simulink model "payment_donation_hcs_2020"  (R2020a)
settings: Solver=VariableStepAuto  StartTime=0.0  StopTime=10.0  RelTol=1e-3
(part 1 of 2)
settings Model: Creator=ayj  LastModifiedBy=ayj
settings DebuggingCC: UnconnectedInputMsg=none  UnconnectedOutputMsg=none  UnconnectedLineMsg=none  SFMachineParentedDataDiag=error

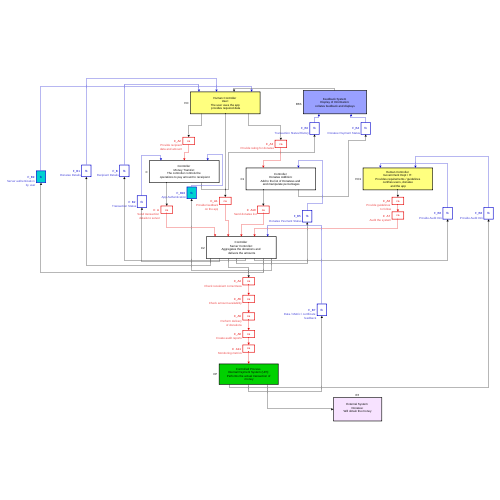
[thumbnail: Simulink's stored preview of the top-level diagram]
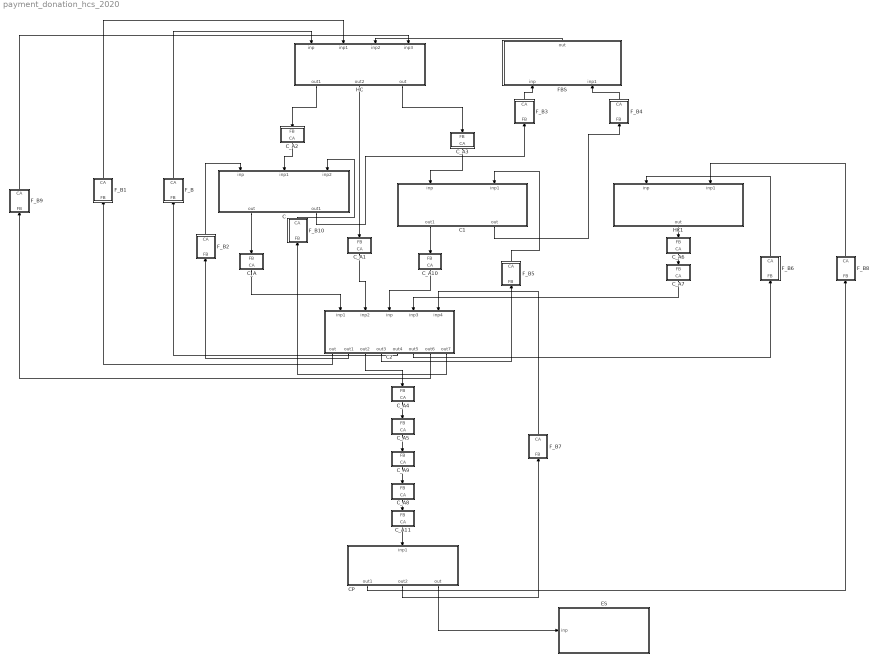
== system payment_donation_hcs_2020 ==
  " FBS" : Subsystem  TreatAsAtomicUnit=on  mask(feedback_system){NAMEFORBLOCK=Display of Information, DES=collates feedback and displays}
      mask prompts: NAMEFORBLOCK "Provide a name"; DES "Provide a description of feedback system"
      mask help: Say what this feedback system does
      mask init:
      | set_param(gcb,'LinkStatus', 'none');
      settings: RTWFcnNameOpts=Use subsystem name  RTWFileNameOpts=Use function name
      mask DialogControl Control2 Prompt: ADD Input
      mask DialogControl Control2 Callback:
      | h = add_block('simulink/Sources/In1', [gcb '/inp'], 'MakeNameUnique', 'on');
      | hg = add_block('simulink/Sinks/Terminator', [gcb '/term'], 'MakeNameUnique', 'on');
      | hname = get_param(h,'PortHandles');
      | hgname = get_param(hg,'PortHandles');
      | add_line(gcb, hname.Outport(1), hgname.Inport(1));
      mask DialogControl Control3 Prompt: ADD Output
      mask DialogControl Control3 Callback:
      | h = add_block('simulink/Sinks/Out1', [gcb '/out'], 'MakeNameUnique', 'on');
      | hg = add_block('simulink/Sources/Ground', [gcb '/gnd'], 'MakeNameUnique', 'on');
      | hname = get_param(h,'PortHandles');
      | hgname = get_param(hg,'PortHandles');
      | add_line(gcb, hgname.Outport(1), hname.Inport(1));
      mask DialogControl Control4 Prompt: REM Input
      mask DialogControl Control4 Callback:
      | a=find_system(gcb,'SearchDepth',2,'LookUnderMasks','all','BlockType','Inport');
      | if ~isempty(a)
      | b=get_param(a{1},'PortConnectivity');
      | delete_block(a{1});
      | delete_block(b.DstBlock);
      | delete_line(find_system(gcb, 'SearchDepth',2,'LookUnderMasks','all','FindAll', 'on', 'Type', 'line', 'Connected', 'off'))
      | end
      mask DialogControl Control5 Prompt: REM Output
      mask DialogControl Control5 Callback:
      | a=find_system(gcb,'SearchDepth',2,'LookUnderMasks','all','BlockType','Outport');
      | if ~isempty(a)
      | b=get_param(a{1},'PortConnectivity');
      | delete_block(a{1});
      | delete_block(b.SrcBlock);
      | delete_line(find_system(gcb, 'SearchDepth',2,'LookUnderMasks','all','FindAll', 'on', 'Type', 'line', 'Connected', 'off'))
      | end
      mask Display: disp(['Feedback System \n' NAMEFORBLOCK ':\n' DES])
  C : Subsystem  TreatAsAtomicUnit=on  mask(controller){NAMEFORBLOCK=Money Transfer, DES=The controller controls the \n operations to pay amount to receipient}
      mask prompts: NAMEFORBLOCK "Provide a name for Block"; DES "Provide a description of Responsibility"
      mask help: Say what this controller does
      mask init:
      | set_param(gcb,'LinkStatus', 'none');
      settings: RTWFcnNameOpts=Use subsystem name  RTWFileNameOpts=Use function name
      mask DialogControl Control2 Prompt: ADD Input
      mask DialogControl Control2 Callback:
      | h = add_block('simulink/Sources/In1', [gcb '/inp'], 'MakeNameUnique', 'on');
      | hg = add_block('simulink/Sinks/Terminator', [gcb '/term'], 'MakeNameUnique', 'on');
      | hname = get_param(h,'PortHandles');
      | hgname = get_param(hg,'PortHandles');
      | add_line(gcb, hname.Outport(1), hgname.Inport(1));
      mask DialogControl Control3 Prompt: ADD Output
      mask DialogControl Control3 Callback:
      | h = add_block('simulink/Sinks/Out1', [gcb '/out'], 'MakeNameUnique', 'on');
      | hg = add_block('simulink/Sources/Ground', [gcb '/gnd'], 'MakeNameUnique', 'on');
      | hname = get_param(h,'PortHandles');
      | hgname = get_param(hg,'PortHandles');
      | add_line(gcb, hgname.Outport(1), hname.Inport(1));
      mask DialogControl Control4 Prompt: REM Input
      mask DialogControl Control4 Callback:
      | a=find_system(gcb,'SearchDepth',2,'LookUnderMasks','all','BlockType','Inport');
      | if ~isempty(a)
      | b=get_param(a{1},'PortConnectivity');
      | delete_block(a{1});
      | delete_block(b.DstBlock);
      | delete_line(find_system(gcb, 'SearchDepth',2,'LookUnderMasks','all','FindAll', 'on', 'Type', 'line', 'Connected', 'off'))
      | end
      mask DialogControl Control5 Prompt: REM Output
      mask DialogControl Control5 Callback:
      | a=find_system(gcb,'SearchDepth',2,'LookUnderMasks','all','BlockType','Outport');
      | if ~isempty(a)
      | b=get_param(a{1},'PortConnectivity');
      | delete_block(a{1});
      | delete_block(b.SrcBlock);
      | delete_line(find_system(gcb, 'SearchDepth',2,'LookUnderMasks','all','FindAll', 'on', 'Type', 'line', 'Connected', 'off'))
      | end
      mask Display: disp(['Controller \n' NAMEFORBLOCK ':\n' DES])
  C1 : Subsystem  TreatAsAtomicUnit=on  mask(controller){NAMEFORBLOCK=Donatee Addition, DES=Add to the list of Donatess and \n and manipulate percentages}
      mask prompts: NAMEFORBLOCK "Provide a name for Block"; DES "Provide a description of Responsibility"
      mask help: Say what this controller does
      mask init:
      | set_param(gcb,'LinkStatus', 'none');
      settings: RTWFcnNameOpts=Use subsystem name  RTWFileNameOpts=Use function name
      mask DialogControl Control2 Prompt: ADD Input
      mask DialogControl Control2 Callback:
      | h = add_block('simulink/Sources/In1', [gcb '/inp'], 'MakeNameUnique', 'on');
      | hg = add_block('simulink/Sinks/Terminator', [gcb '/term'], 'MakeNameUnique', 'on');
      | hname = get_param(h,'PortHandles');
      | hgname = get_param(hg,'PortHandles');
      | add_line(gcb, hname.Outport(1), hgname.Inport(1));
      mask DialogControl Control3 Prompt: ADD Output
      mask DialogControl Control3 Callback:
      | h = add_block('simulink/Sinks/Out1', [gcb '/out'], 'MakeNameUnique', 'on');
      | hg = add_block('simulink/Sources/Ground', [gcb '/gnd'], 'MakeNameUnique', 'on');
      | hname = get_param(h,'PortHandles');
      | hgname = get_param(hg,'PortHandles');
      | add_line(gcb, hgname.Outport(1), hname.Inport(1));
      mask DialogControl Control4 Prompt: REM Input
      mask DialogControl Control4 Callback:
      | a=find_system(gcb,'SearchDepth',2,'LookUnderMasks','all','BlockType','Inport');
      | if ~isempty(a)
      | b=get_param(a{1},'PortConnectivity');
      | delete_block(a{1});
      | delete_block(b.DstBlock);
      | delete_line(find_system(gcb, 'SearchDepth',2,'LookUnderMasks','all','FindAll', 'on', 'Type', 'line', 'Connected', 'off'))
      | end
      mask DialogControl Control5 Prompt: REM Output
      mask DialogControl Control5 Callback:
      | a=find_system(gcb,'SearchDepth',2,'LookUnderMasks','all','BlockType','Outport');
      | if ~isempty(a)
      | b=get_param(a{1},'PortConnectivity');
      | delete_block(a{1});
      | delete_block(b.SrcBlock);
      | delete_line(find_system(gcb, 'SearchDepth',2,'LookUnderMasks','all','FindAll', 'on', 'Type', 'line', 'Connected', 'off'))
      | end
      mask Display: disp(['Controller \n' NAMEFORBLOCK ':\n' DES])
  C2 : Subsystem  TreatAsAtomicUnit=on  mask(controller){NAMEFORBLOCK=Server Controller, DES=Aggregates the donations and \n delivers the amounts}
      mask prompts: NAMEFORBLOCK "Provide a name for Block"; DES "Provide a description of Responsibility"
      mask help: Say what this controller does
      mask init:
      | set_param(gcb,'LinkStatus', 'none');
      settings: RTWFcnNameOpts=Use subsystem name  RTWFileNameOpts=Use function name
      mask DialogControl Control2 Prompt: ADD Input
      mask DialogControl Control2 Callback:
      | h = add_block('simulink/Sources/In1', [gcb '/inp'], 'MakeNameUnique', 'on');
      | hg = add_block('simulink/Sinks/Terminator', [gcb '/term'], 'MakeNameUnique', 'on');
      | hname = get_param(h,'PortHandles');
      | hgname = get_param(hg,'PortHandles');
      | add_line(gcb, hname.Outport(1), hgname.Inport(1));
      mask DialogControl Control3 Prompt: ADD Output
      mask DialogControl Control3 Callback:
      | h = add_block('simulink/Sinks/Out1', [gcb '/out'], 'MakeNameUnique', 'on');
      | hg = add_block('simulink/Sources/Ground', [gcb '/gnd'], 'MakeNameUnique', 'on');
      | hname = get_param(h,'PortHandles');
      | hgname = get_param(hg,'PortHandles');
      | add_line(gcb, hgname.Outport(1), hname.Inport(1));
      mask DialogControl Control4 Prompt: REM Input
      mask DialogControl Control4 Callback:
      | a=find_system(gcb,'SearchDepth',2,'LookUnderMasks','all','BlockType','Inport');
      | if ~isempty(a)
      | b=get_param(a{1},'PortConnectivity');
      | delete_block(a{1});
      | delete_block(b.DstBlock);
      | delete_line(find_system(gcb, 'SearchDepth',2,'LookUnderMasks','all','FindAll', 'on', 'Type', 'line', 'Connected', 'off'))
      | end
      mask DialogControl Control5 Prompt: REM Output
      mask DialogControl Control5 Callback:
      | a=find_system(gcb,'SearchDepth',2,'LookUnderMasks','all','BlockType','Outport');
      | if ~isempty(a)
      | b=get_param(a{1},'PortConnectivity');
      | delete_block(a{1});
      | delete_block(b.SrcBlock);
      | delete_line(find_system(gcb, 'SearchDepth',2,'LookUnderMasks','all','FindAll', 'on', 'Type', 'line', 'Connected', 'off'))
      | end
      mask Display: disp(['Controller \n' NAMEFORBLOCK ':\n' DES])
  CP : Subsystem  TreatAsAtomicUnit=on  mask(controlled_process){NAMEFORBLOCK=Internal Payment System (UPI), DES=Performs the actual transaction of\n money}
      mask prompts: NAMEFORBLOCK "Provide a name for Block"; DES "Provide a description of Responsibility"
      mask help: Say what this controlled process does
      settings: RTWFcnNameOpts=Use subsystem name  RTWFileNameOpts=Use function name
      mask DialogControl Control2 Prompt: ADD Input
      mask DialogControl Control2 Callback:
      | set_param(gcb,'LinkStatus', 'none');
      | h = add_block('simulink/Sources/In1', [gcb '/inp'], 'MakeNameUnique', 'on');
      | hg = add_block('simulink/Sinks/Terminator', [gcb '/term'], 'MakeNameUnique', 'on');
      | hname = get_param(h,'PortHandles');
      | hgname = get_param(hg,'PortHandles');
      | add_line(gcb, hname.Outport(1), hgname.Inport(1));
      mask DialogControl Control3 Prompt: ADD Output
      mask DialogControl Control3 Callback:
      | set_param(gcb,'LinkStatus', 'none');
      | h = add_block('simulink/Sinks/Out1', [gcb '/out'], 'MakeNameUnique', 'on');
      | hg = add_block('simulink/Sources/Ground', [gcb '/gnd'], 'MakeNameUnique', 'on');
      | hname = get_param(h,'PortHandles');
      | hgname = get_param(hg,'PortHandles');
      | add_line(gcb, hgname.Outport(1), hname.Inport(1));
      mask DialogControl Control4 Prompt: REM Input
      mask DialogControl Control4 Callback:
      | set_param(gcb,'LinkStatus', 'none');
      | a=find_system(gcb,'SearchDepth',2,'LookUnderMasks','all','BlockType','Inport');
      | if ~isempty(a)
      | b=get_param(a{1},'PortConnectivity');
      | delete_block(a{1});
      | delete_block(b.DstBlock);
      | delete_line(find_system(gcb, 'SearchDepth',2,'LookUnderMasks','all','FindAll', 'on', 'Type', 'line', 'Connected', 'off'))
      | end
      mask DialogControl Control5 Prompt: REM Output
      mask DialogControl Control5 Callback:
      | set_param(gcb,'LinkStatus', 'none');
      | a=find_system(gcb,'SearchDepth',2,'LookUnderMasks','all','BlockType','Outport');
      | if ~isempty(a)
      | b=get_param(a{1},'PortConnectivity');
      | delete_block(a{1});
      | delete_block(b.SrcBlock);
      | delete_line(find_system(gcb, 'SearchDepth',2,'LookUnderMasks','all','FindAll', 'on', 'Type', 'line', 'Connected', 'off'))
      | end
      mask Display: disp(['Controlled Process \n' NAMEFORBLOCK ':\n' DES])
  C_A : Subsystem  TreatAsAtomicUnit=on  mask(control_action){DES=Send transaction \ndetails to server, UCA1=[#H6][#H5] Not providing the request for transaction, UCA2=[#H1][#H2][#H6] Providing incorrect/unauthorised data to server, UCA3=[#H6][#H5] Providing request late or early without authorisation, UCA4=[#H6] Continuously send request, or stop request too soon}
      mask prompts: DES "Provide a description of Control Action"; UCA1 "Not providing causes hazard [link Hazard]"; UCA2 "Providing causes hazard [link Hazard]"; UCA3 "Too early, too late, out of order [link Hazard]"; UCA4 "Stopped too soon, applied too long [link Hazard]"
      mask help:
      | <Source> <Type> <Control Action> <Context> <Link to Hazards>
      | Source = System Above, Type = {provided, not provided ..], Control Action = command
      | from the description, Context = While/When .. Always link to a hazard
      mask init:
      | set_param(gcb,'LinkStatus', 'none');
      settings: AttributesFormatString=%<DES>  RTWFcnNameOpts=Use subsystem name  RTWFileNameOpts=Use function name
      mask Display: disp('ca')
  C_A1 : Subsystem  TreatAsAtomicUnit=on  mask(control_action){DES=Provide feedback\n on the app, UCA1=[#H5] Not providing any issues with app, UCA2=[#H5] Providing wrong feedback on the app, UCA3=[#H5] Providing feedback on old issues already fixed, UCA4=[#H5] Providing the same feedback on realised issue}
      mask prompts: DES "Provide a description of Control Action"; UCA1 "Not providing causes hazard [link Hazard]"; UCA2 "Providing causes hazard [link Hazard]"; UCA3 "Too early, too late, out of order [link Hazard]"; UCA4 "Stopped too soon, applied too long [link Hazard]"
      mask help:
      | <Source> <Type> <Control Action> <Context> <Link to Hazards>
      | Source = System Above, Type = {provided, not provided ..], Control Action = command
      | from the description, Context = While/When .. Always link to a hazard
      mask init:
      | set_param(gcb,'LinkStatus', 'none');
      settings: AttributesFormatString=%<DES>  RTWFcnNameOpts=Use subsystem name  RTWFileNameOpts=Use function name
      mask Display: disp('ca')
  C_A10 : Subsystem  TreatAsAtomicUnit=on  mask(control_action){DES=Send donatee list, UCA1=[#H5][#H4] Not providing list approved by user, UCA2=[#H4][#H5] Providing a list not approved by the user, UCA3=[#H6][#H5] Providing donatee list too late after user approves, UCA4=[#H5] Updated donatee list not refreshed/old list continuously sent}
      mask prompts: DES "Provide a description of Control Action"; UCA1 "Not providing causes hazard [link Hazard]"; UCA2 "Providing causes hazard [link Hazard]"; UCA3 "Too early, too late, out of order [link Hazard]"; UCA4 "Stopped too soon, applied too long [link Hazard]"
      mask help:
      | <Source> <Type> <Control Action> <Context> <Link to Hazards>
      | Source = System Above, Type = {provided, not provided ..], Control Action = command
      | from the description, Context = While/When .. Always link to a hazard
      mask init:
      | set_param(gcb,'LinkStatus', 'none');
      settings: AttributesFormatString=%<DES>  RTWFcnNameOpts=Use subsystem name  RTWFileNameOpts=Use function name
      mask Display: disp('ca')
  C_A11 : Subsystem  TreatAsAtomicUnit=on  mask(control_action){DES=Monitoring metrics, UCA1=[#H5][#H3] Not providing metrics for app improvement, UCA2=, UCA3=[#H5] Providing metrics too late, UCA4=}
      mask prompts: DES "Provide a description of Control Action"; UCA1 "Not providing causes hazard [link Hazard]"; UCA2 "Providing causes hazard [link Hazard]"; UCA3 "Too early, too late, out of order [link Hazard]"; UCA4 "Stopped too soon, applied too long [link Hazard]"
      mask help:
      | <Source> <Type> <Control Action> <Context> <Link to Hazards>
      | Source = System Above, Type = {provided, not provided ..], Control Action = command
      | from the description, Context = While/When .. Always link to a hazard
      mask init:
      | set_param(gcb,'LinkStatus', 'none');
      settings: AttributesFormatString=%<DES>  RTWFcnNameOpts=Use subsystem name  RTWFileNameOpts=Use function name
      mask Display: disp('ca')
  C_A2 : Subsystem  TreatAsAtomicUnit=on  mask(control_action){DES=Provide recipient\n data and amount, UCA1=[#H5] Not providing data in the app, UCA2=[#H1][#H2] Providing incorrect data, UCA3=[#H6] Providing data when unpromted, UCA4=[#H6] Stopped data entry too soon (scanning quickly)}
      mask prompts: DES "Provide a description of Control Action"; UCA1 "Not providing causes hazard [link Hazard]"; UCA2 "Providing causes hazard [link Hazard]"; UCA3 "Too early, too late, out of order [link Hazard]"; UCA4 "Stopped too soon, applied too long [link Hazard]"
      mask help:
      | <Source> <Type> <Control Action> <Context> <Link to Hazards>
      | Source = System Above, Type = {provided, not provided ..], Control Action = command
      | from the description, Context = While/When .. Always link to a hazard
      mask init:
      | set_param(gcb,'LinkStatus', 'none');
      settings: AttributesFormatString=%<DES>  RTWFcnNameOpts=Use subsystem name  RTWFileNameOpts=Use function name
      mask Display: disp('ca')
  C_A3 : Subsystem  TreatAsAtomicUnit=on  mask(control_action){DES=Provide rating for donatee, UCA1=[#H4][#H5] Not providing details of bad donatee, UCA2=[#H5] Providing wrong feedback for donatee, UCA3=[#H4] Providing feedback late and list late, UCA4=[#H4][#H3] providing donatee list and removing within month}
      mask prompts: DES "Provide a description of Control Action"; UCA1 "Not providing causes hazard [link Hazard]"; UCA2 "Providing causes hazard [link Hazard]"; UCA3 "Too early, too late, out of order [link Hazard]"; UCA4 "Stopped too soon, applied too long [link Hazard]"
      mask help:
      | <Source> <Type> <Control Action> <Context> <Link to Hazards>
      | Source = System Above, Type = {provided, not provided ..], Control Action = command
      | from the description, Context = While/When .. Always link to a hazard
      mask init:
      | set_param(gcb,'LinkStatus', 'none');
      settings: AttributesFormatString=%<DES>  RTWFcnNameOpts=Use subsystem name  RTWFileNameOpts=Use function name
      mask Display: disp('ca')
  C_A4 : Subsystem  TreatAsAtomicUnit=on  mask(control_action){DES=Check receipient correctness, UCA1=[#H1] Not checking the correct recipient, UCA2=[#H1] Providing a check for incorrect recipient, UCA3=[#H6][#H1] Checking the recipient requests out of order, UCA4=[#H6] Request for check timed out or stopped too soon}
      mask prompts: DES "Provide a description of Control Action"; UCA1 "Not providing causes hazard [link Hazard]"; UCA2 "Providing causes hazard [link Hazard]"; UCA3 "Too early, too late, out of order [link Hazard]"; UCA4 "Stopped too soon, applied too long [link Hazard]"
      mask help:
      | <Source> <Type> <Control Action> <Context> <Link to Hazards>
      | Source = System Above, Type = {provided, not provided ..], Control Action = command
      | from the description, Context = While/When .. Always link to a hazard
      mask init:
      | set_param(gcb,'LinkStatus', 'none');
      settings: AttributesFormatString=%<DES>  RTWFcnNameOpts=Use subsystem name  RTWFileNameOpts=Use function name
      mask Display: disp('ca')
  C_A5 : Subsystem  TreatAsAtomicUnit=on  mask(control_action){DES=Check amount availability, UCA1=[#H6][#H2] Not providing check for balance before withdraw, UCA2=[#H6][#H2] Providing wrong check for balance, UCA3=[#H6][#H2] Providing check too late, out of order, UCA4=[#H6][#H2] Providing check of balance too late}
      mask prompts: DES "Provide a description of Control Action"; UCA1 "Not providing causes hazard [link Hazard]"; UCA2 "Providing causes hazard [link Hazard]"; UCA3 "Too early, too late, out of order [link Hazard]"; UCA4 "Stopped too soon, applied too long [link Hazard]"
      mask help:
      | <Source> <Type> <Control Action> <Context> <Link to Hazards>
      | Source = System Above, Type = {provided, not provided ..], Control Action = command
      | from the description, Context = While/When .. Always link to a hazard
      mask init:
      | set_param(gcb,'LinkStatus', 'none');
      settings: AttributesFormatString=%<DES>  RTWFcnNameOpts=Use subsystem name  RTWFileNameOpts=Use function name
      mask Display: disp('ca')
  C_A6 : Subsystem  TreatAsAtomicUnit=on  mask(control_action){DES=Provide guidelines \nto follow, UCA1=[#H3][#H5] Not providing guidelines to follow, UCA2=, UCA3=[#H3] Providing guidelines too late, UCA4=}
      mask prompts: DES "Provide a description of Control Action"; UCA1 "Not providing causes hazard [link Hazard]"; UCA2 "Providing causes hazard [link Hazard]"; UCA3 "Too early, too late, out of order [link Hazard]"; UCA4 "Stopped too soon, applied too long [link Hazard]"
      mask help:
      | <Source> <Type> <Control Action> <Context> <Link to Hazards>
      | Source = System Above, Type = {provided, not provided ..], Control Action = command
      | from the description, Context = While/When .. Always link to a hazard
      mask init:
      | set_param(gcb,'LinkStatus', 'none');
      settings: AttributesFormatString=%<DES>  RTWFcnNameOpts=Use subsystem name  RTWFileNameOpts=Use function name
      mask Display: disp('ca')
  C_A7 : Subsystem  TreatAsAtomicUnit=on  mask(control_action){DES=Audit the system, UCA1=[#H3][#H5] Not providing audits of system, UCA2=[#H6] Providing audits which affect business processes, UCA3=[#H3] providing audit too late, UCA4=}
      mask prompts: DES "Provide a description of Control Action"; UCA1 "Not providing causes hazard [link Hazard]"; UCA2 "Providing causes hazard [link Hazard]"; UCA3 "Too early, too late, out of order [link Hazard]"; UCA4 "Stopped too soon, applied too long [link Hazard]"
      mask help:
      | <Source> <Type> <Control Action> <Context> <Link to Hazards>
      | Source = System Above, Type = {provided, not provided ..], Control Action = command
      | from the description, Context = While/When .. Always link to a hazard
      mask init:
      | set_param(gcb,'LinkStatus', 'none');
      settings: AttributesFormatString=%<DES>  RTWFcnNameOpts=Use subsystem name  RTWFileNameOpts=Use function name
      mask Display: disp('ca')
  C_A8 : Subsystem  TreatAsAtomicUnit=on  mask(control_action){DES=Create audit reports, UCA1=[#H3] Not providing audit reports for analysis, UCA2=[#H3] Providing incorrect audit report, UCA3=[#H3] Providing reports too late, UCA4=}
      mask prompts: DES "Provide a description of Control Action"; UCA1 "Not providing causes hazard [link Hazard]"; UCA2 "Providing causes hazard [link Hazard]"; UCA3 "Too early, too late, out of order [link Hazard]"; UCA4 "Stopped too soon, applied too long [link Hazard]"
      mask help:
      | <Source> <Type> <Control Action> <Context> <Link to Hazards>
      | Source = System Above, Type = {provided, not provided ..], Control Action = command
      | from the description, Context = While/When .. Always link to a hazard
      mask init:
      | set_param(gcb,'LinkStatus', 'none');
      settings: AttributesFormatString=%<DES>  RTWFcnNameOpts=Use subsystem name  RTWFileNameOpts=Use function name
      mask Display: disp('ca')
  C_A9 : Subsystem  TreatAsAtomicUnit=on  mask(control_action){DES=Perform delivery\n of donations, UCA1=[#H3][#H5] Not providing donation money to donatees, UCA2=[#H5][#H4] Money provided to wrong donatees, or more than once, UCA3=[#H5][#H6] Donation money provided too late/without enough balance, UCA4=[#H4][#H5][#H2] Donation money provided to old donatees without updation}
      mask prompts: DES "Provide a description of Control Action"; UCA1 "Not providing causes hazard [link Hazard]"; UCA2 "Providing causes hazard [link Hazard]"; UCA3 "Too early, too late, out of order [link Hazard]"; UCA4 "Stopped too soon, applied too long [link Hazard]"
      mask help:
      | <Source> <Type> <Control Action> <Context> <Link to Hazards>
      | Source = System Above, Type = {provided, not provided ..], Control Action = command
      | from the description, Context = While/When .. Always link to a hazard
      mask init:
      | set_param(gcb,'LinkStatus', 'none');
      settings: AttributesFormatString=%<DES>  RTWFcnNameOpts=Use subsystem name  RTWFileNameOpts=Use function name
      mask Display: disp('ca')
  ES : Subsystem  TreatAsAtomicUnit=on  mask(external_system){NAMEFORBLOCK=Donatee, DES=Will obtain the money\n}
      mask prompts: NAMEFORBLOCK "Provide a name for Block"; DES "Provide a description of the Interaction"
      mask help: Say how this external system interacts with the process
      mask init:
      | set_param(gcb,'LinkStatus', 'none');
      settings: RTWFcnNameOpts=Use subsystem name  RTWFileNameOpts=Use function name
      mask DialogControl Control2 Prompt: ADD Input
      mask DialogControl Control2 Callback:
      | h = add_block('simulink/Sources/In1', [gcb '/inp'], 'MakeNameUnique', 'on');
      | hg = add_block('simulink/Sinks/Terminator', [gcb '/term'], 'MakeNameUnique', 'on');
      | hname = get_param(h,'PortHandles');
      | hgname = get_param(hg,'PortHandles');
      | add_line(gcb, hname.Outport(1), hgname.Inport(1));
      mask DialogControl Control3 Prompt: ADD Output
      mask DialogControl Control3 Callback:
      | h = add_block('simulink/Sinks/Out1', [gcb '/out'], 'MakeNameUnique', 'on');
      | hg = add_block('simulink/Sources/Ground', [gcb '/gnd'], 'MakeNameUnique', 'on');
      | hname = get_param(h,'PortHandles');
      | hgname = get_param(hg,'PortHandles');
      | add_line(gcb, hgname.Outport(1), hname.Inport(1));
      mask DialogControl Control4 Prompt: REM Input
      mask DialogControl Control4 Callback:
      | a=find_system(gcb,'SearchDepth',2,'LookUnderMasks','all','BlockType','Inport');
      | if ~isempty(a)
      | b=get_param(a{1},'PortConnectivity');
      | delete_block(a{1});
      | delete_block(b.DstBlock);
      | delete_line(find_system(gcb, 'SearchDepth',2,'LookUnderMasks','all','FindAll', 'on', 'Type', 'line', 'Connected', 'off'))
      | end
      mask DialogControl Control5 Prompt: REM Output
      mask DialogControl Control5 Callback:
      | a=find_system(gcb,'SearchDepth',2,'LookUnderMasks','all','BlockType','Outport');
      | if ~isempty(a)
      | b=get_param(a{1},'PortConnectivity');
      | delete_block(a{1});
      | delete_block(b.SrcBlock);
      | delete_line(find_system(gcb, 'SearchDepth',2,'LookUnderMasks','all','FindAll', 'on', 'Type', 'line', 'Connected', 'off'))
      | end
      mask Display: disp(['External System \n' NAMEFORBLOCK ':\n' DES])
  F_B : Subsystem  TreatAsAtomicUnit=on  mask(feedback){DES=Recipient Details}
      mask prompts: DES "Provide a description"
      mask help: Say what this feeds back from the system
      mask init:
      | set_param(gcb,'LinkStatus', 'none');
      settings: AttributesFormatString=%<DES>  RTWFcnNameOpts=Use subsystem name  RTWFileNameOpts=Use function name
      mask Display: disp('fb')
  F_B1 : Subsystem  TreatAsAtomicUnit=on  mask(feedback){DES=Donatee Details}
      mask prompts: DES "Provide a description"
      mask help: Say what this feeds back from the system
      mask init:
      | set_param(gcb,'LinkStatus', 'none');
      settings: AttributesFormatString=%<DES>  RTWFcnNameOpts=Use subsystem name  RTWFileNameOpts=Use function name
      mask Display: disp('fb')
  F_B10 : Subsystem  TreatAsAtomicUnit=on  mask(feedback){DES=App Authentication}
      mask prompts: DES "Provide a description"
      mask help: Say what this feeds back from the system
      mask init:
      | set_param(gcb,'LinkStatus', 'none');
      settings: AttributesFormatString=%<DES>  RTWFcnNameOpts=Use subsystem name  RTWFileNameOpts=Use function name
      mask Display: disp('fb')
  F_B2 : Subsystem  TreatAsAtomicUnit=on  mask(feedback){DES=Transaction Status}
      mask prompts: DES "Provide a description"
      mask help: Say what this feeds back from the system
      mask init:
      | set_param(gcb,'LinkStatus', 'none');
      settings: AttributesFormatString=%<DES>  RTWFcnNameOpts=Use subsystem name  RTWFileNameOpts=Use function name
      mask Display: disp('fb')
  F_B3 : Subsystem  TreatAsAtomicUnit=on  mask(feedback){DES=Transaction Status/History}
      mask prompts: DES "Provide a description"
      mask help: Say what this feeds back from the system
      mask init:
      | set_param(gcb,'LinkStatus', 'none');
      settings: AttributesFormatString=%<DES>  RTWFcnNameOpts=Use subsystem name  RTWFileNameOpts=Use function name
      mask Display: disp('fb')
  F_B4 : Subsystem  TreatAsAtomicUnit=on  mask(feedback){DES=Donatee Payment Status}
      mask prompts: DES "Provide a description"
      mask help: Say what this feeds back from the system
      mask init:
      | set_param(gcb,'LinkStatus', 'none');
      settings: AttributesFormatString=%<DES>  RTWFcnNameOpts=Use subsystem name  RTWFileNameOpts=Use function name
      mask Display: disp('fb')
  F_B5 : Subsystem  TreatAsAtomicUnit=on  mask(feedback){DES=Donatee Payment Status}
      mask prompts: DES "Provide a description"
      mask help: Say what this feeds back from the system
      mask init:
      | set_param(gcb,'LinkStatus', 'none');
      settings: AttributesFormatString=%<DES>  RTWFcnNameOpts=Use subsystem name  RTWFileNameOpts=Use function name
      mask Display: disp('fb')
  F_B6 : Subsystem  TreatAsAtomicUnit=on  mask(feedback){DES=Provide Audit Info}
      mask prompts: DES "Provide a description"
      mask help: Say what this feeds back from the system
      mask init:
      | set_param(gcb,'LinkStatus', 'none');
      settings: AttributesFormatString=%<DES>  RTWFcnNameOpts=Use subsystem name  RTWFileNameOpts=Use function name
      mask Display: disp('fb')
  F_B7 : Subsystem  TreatAsAtomicUnit=on  mask(feedback){DES=Data / Metric / certificate \n feedback}
      mask prompts: DES "Provide a description"
      mask help: Say what this feeds back from the system
      mask init:
      | set_param(gcb,'LinkStatus', 'none');
      settings: AttributesFormatString=%<DES>  RTWFcnNameOpts=Use subsystem name  RTWFileNameOpts=Use function name
      mask Display: disp('fb')
  F_B8 : Subsystem  TreatAsAtomicUnit=on  mask(feedback){DES=Provide Audit Info}
      mask prompts: DES "Provide a description"
      mask help: Say what this feeds back from the system
      mask init:
      | set_param(gcb,'LinkStatus', 'none');
      settings: AttributesFormatString=%<DES>  RTWFcnNameOpts=Use subsystem name  RTWFileNameOpts=Use function name
      mask Display: disp('fb')
  F_B9 : Subsystem  TreatAsAtomicUnit=on  mask(feedback){DES=Server authentication \n by user}
      mask prompts: DES "Provide a description"
      mask help: Say what this feeds back from the system
      mask init:
      | set_param(gcb,'LinkStatus', 'none');
      settings: AttributesFormatString=%<DES>  RTWFcnNameOpts=Use subsystem name  RTWFileNameOpts=Use function name
      mask Display: disp('fb')
  HC : Subsystem  TreatAsAtomicUnit=on  mask(human_controller){NAMEFORBLOCK=User, DES=The user uses the app\n provides required data}
      mask prompts: NAMEFORBLOCK "Provide a name for Block"; DES "Provide a description of Responsibility"
      mask help: Say what this human controller does
      mask init:
      | set_param(gcb,'LinkStatus','none')
      settings: RTWFcnNameOpts=Use subsystem name  RTWFileNameOpts=Use function name
      mask DialogControl Control2 Prompt: ADD Input
      mask DialogControl Control2 Callback:
      | h = add_block('simulink/Sources/In1', [gcb '/inp'], 'MakeNameUnique', 'on');
      | hg = add_block('simulink/Sinks/Terminator', [gcb '/term'], 'MakeNameUnique', 'on');
      | hname = get_param(h,'PortHandles');
      | hgname = get_param(hg,'PortHandles');
      | add_line(gcb, hname.Outport(1), hgname.Inport(1));
      mask DialogControl Control3 Prompt: ADD Output
      mask DialogControl Control3 Callback:
      | h = add_block('simulink/Sinks/Out1', [gcb '/out'], 'MakeNameUnique', 'on');
      | hg = add_block('simulink/Sources/Ground', [gcb '/gnd'], 'MakeNameUnique', 'on');
      | hname = get_param(h,'PortHandles');
      | hgname = get_param(hg,'PortHandles');
      | add_line(gcb, hgname.Outport(1), hname.Inport(1));
      mask DialogControl Control4 Prompt: REM Input
      mask DialogControl Control4 Callback:
      | a=find_system(gcb,'SearchDepth',2,'LookUnderMasks','all','BlockType','Inport');
      | if ~isempty(a)
      | b=get_param(a{1},'PortConnectivity');
      | delete_block(a{1});
      | delete_block(b.DstBlock);
      | delete_line(find_system(gcb, 'SearchDepth',2,'LookUnderMasks','all','FindAll', 'on', 'Type', 'line', 'Connected', 'off'))
      | end
      mask DialogControl Control5 Prompt: REM Output
      mask DialogControl Control5 Callback:
      | a=find_system(gcb,'SearchDepth',2,'LookUnderMasks','all','BlockType','Outport');
      | if ~isempty(a)
      | b=get_param(a{1},'PortConnectivity');
      | delete_block(a{1});
      | delete_block(b.SrcBlock);
      | delete_line(find_system(gcb, 'SearchDepth',2,'LookUnderMasks','all','FindAll', 'on', 'Type', 'line', 'Connected', 'off'))
      | end
      mask Display: disp(['Human Controller \n' NAMEFORBLOCK ':\n' DES])
  HC1 : Subsystem  TreatAsAtomicUnit=on  mask(human_controller){NAMEFORBLOCK=Government Dept / IT, DES=Provides requirements / guidelines\ncertifies users, donatee\n and the app}
      mask prompts: NAMEFORBLOCK "Provide a name for Block"; DES "Provide a description of Responsibility"
      mask help: Say what this human controller does
      mask init:
      | set_param(gcb,'LinkStatus','none')
      settings: RTWFcnNameOpts=Use subsystem name  RTWFileNameOpts=Use function name
      mask DialogControl Control2 Prompt: ADD Input
      mask DialogControl Control2 Callback:
      | h = add_block('simulink/Sources/In1', [gcb '/inp'], 'MakeNameUnique', 'on');
      | hg = add_block('simulink/Sinks/Terminator', [gcb '/term'], 'MakeNameUnique', 'on');
      | hname = get_param(h,'PortHandles');
      | hgname = get_param(hg,'PortHandles');
      | add_line(gcb, hname.Outport(1), hgname.Inport(1));
      mask DialogControl Control3 Prompt: ADD Output
      mask DialogControl Control3 Callback:
      | h = add_block('simulink/Sinks/Out1', [gcb '/out'], 'MakeNameUnique', 'on');
      | hg = add_block('simulink/Sources/Ground', [gcb '/gnd'], 'MakeNameUnique', 'on');
      | hname = get_param(h,'PortHandles');
      | hgname = get_param(hg,'PortHandles');
      | add_line(gcb, hgname.Outport(1), hname.Inport(1));
      mask DialogControl Control4 Prompt: REM Input
      mask DialogControl Control4 Callback:
      | a=find_system(gcb,'SearchDepth',2,'LookUnderMasks','all','BlockType','Inport');
      | if ~isempty(a)
      | b=get_param(a{1},'PortConnectivity');
      | delete_block(a{1});
      | delete_block(b.DstBlock);
      | delete_line(find_system(gcb, 'SearchDepth',2,'LookUnderMasks','all','FindAll', 'on', 'Type', 'line', 'Connected', 'off'))
      | end
      mask DialogControl Control5 Prompt: REM Output
      mask DialogControl Control5 Callback:
      | a=find_system(gcb,'SearchDepth',2,'LookUnderMasks','all','BlockType','Outport');
      | if ~isempty(a)
      | b=get_param(a{1},'PortConnectivity');
      | delete_block(a{1});
      | delete_block(b.SrcBlock);
      | delete_line(find_system(gcb, 'SearchDepth',2,'LookUnderMasks','all','FindAll', 'on', 'Type', 'line', 'Connected', 'off'))
      | end
      mask Display: disp(['Human Controller \n' NAMEFORBLOCK ':\n' DES])
  wires:
  HC/1(out1) -> C_A2/1(FB)
  HC/3(out) -> C_A3/1(FB)
  C/1(out) -> C_A/1(FB)
  HC1/1(out) -> C_A6/1(FB)
  C1/1(out1) -> C_A10/1(FB)
  C_A/1(CA) -> C2/1(inp1)
  C2/3(out2) -> C_A4/1(FB)
  HC/2(out2) -> C_A1/1(FB)
  C_A2/1(CA) -> C/2(inp1)
  C_A3/1(CA) -> C1/1(inp)
  C_A1/1(CA) -> C2/2(inp2)
  C_A4/1(CA) -> C_A5/1(FB)
  C_A5/1(CA) -> C_A9/1(FB)
  C_A6/1(CA) -> C_A7/1(FB)
  C_A7/1(CA) -> C2/4(inp3)
  C_A9/1(CA) -> C_A8/1(FB)
  C_A10/1(CA) -> C2/3(inp)
  C_A8/1(CA) -> C_A11/1(FB)
  C_A11/1(CA) -> CP/1(inp1)
  C2/5(out4) -> F_B/1(FB)
  F_B/1(CA) -> HC/1(inp)
  F_B1/1(CA) -> HC/2(inp1)
  C2/1(out) -> F_B1/1(FB)
  C2/2(out1) -> F_B2/1(FB)
  F_B2/1(CA) -> C/1(inp)
  F_B3/1(CA) -> " FBS"/1(inp)
  C1/2(out) -> F_B4/1(FB)
  F_B4/1(CA) -> " FBS"/2(inp1)
  C/2(out1) -> F_B3/1(FB)
  " FBS"/1(out) -> HC/3(inp2)
  C2/4(out3) -> F_B5/1(FB)
  F_B5/1(CA) -> C1/2(inp1)
  F_B6/1(CA) -> HC1/1(inp)
  C2/6(out5) -> F_B6/1(FB)
  CP/2(out2) -> F_B7/1(FB)
  F_B7/1(CA) -> C2/5(inp4)
  CP/1(out1) -> F_B8/1(FB)
  F_B8/1(CA) -> HC1/2(inp1)
  CP/3(out) -> ES/1(inp)
  C2/7(out6) -> F_B9/1(FB)
  F_B9/1(CA) -> HC/4(inp3)
  C2/8(out7) -> F_B10/1(FB)
  F_B10/1(CA) -> C/3(inp2)

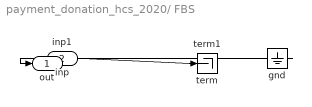
== system payment_donation_hcs_2020/ FBS ==
  inp : Inport
  inp1 : Inport  Port=2
  gnd : Ground
  term : Terminator
  term1 : Terminator
  out : Outport
  wires:
  inp/1 -> term/1
  gnd/1 -> out/1
  inp1/1 -> term1/1

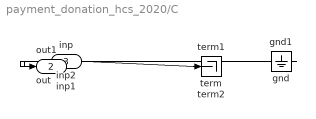
== system payment_donation_hcs_2020/C ==
  inp : Inport
  inp1 : Inport  Port=2
  inp2 : Inport  Port=3
  gnd : Ground
  gnd1 : Ground
  term : Terminator
  term1 : Terminator
  term2 : Terminator
  out : Outport
  out1 : Outport  Port=2
  wires:
  inp/1 -> term/1
  gnd/1 -> out/1
  inp1/1 -> term1/1
  gnd1/1 -> out1/1
  inp2/1 -> term2/1

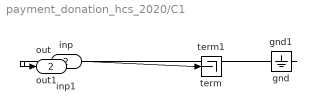
== system payment_donation_hcs_2020/C1 ==
  inp : Inport
  inp1 : Inport  Port=2
  gnd : Ground
  gnd1 : Ground
  term : Terminator
  term1 : Terminator
  out1 : Outport
  out : Outport  Port=2
  wires:
  inp/1 -> term/1
  gnd1/1 -> out1/1
  gnd/1 -> out/1
  inp1/1 -> term1/1

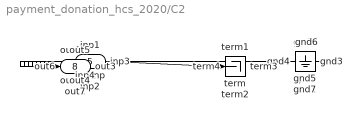
== system payment_donation_hcs_2020/C2 ==
  inp1 : Inport
  inp2 : Inport  Port=2
  inp : Inport  Port=3
  inp3 : Inport  Port=4
  inp4 : Inport  Port=5
  gnd{,1..7} (8 alike) : Ground
  term{,1..4} (5 alike) : Terminator
  out : Outport
  out1 : Outport  Port=2
  out2 : Outport  Port=3
  out3 : Outport  Port=4
  out4 : Outport  Port=5
  out5 : Outport  Port=6
  out6 : Outport  Port=7
  out7 : Outport  Port=8
  wires:
  gnd/1 -> out/1
  inp1/1 -> term1/1
  inp2/1 -> term2/1
  inp/1 -> term/1
  inp3/1 -> term3/1
  gnd1/1 -> out1/1
  gnd2/1 -> out2/1
  gnd3/1 -> out3/1
  gnd4/1 -> out4/1
  gnd5/1 -> out5/1
  inp4/1 -> term4/1
  gnd6/1 -> out6/1
  gnd7/1 -> out7/1

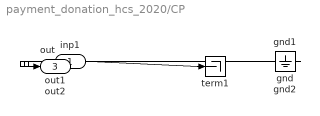
== system payment_donation_hcs_2020/CP ==
  inp1 : Inport
  gnd : Ground
  gnd1 : Ground
  gnd2 : Ground
  term1 : Terminator
  out1 : Outport
  out2 : Outport  Port=2
  out : Outport  Port=3
  wires:
  inp1/1 -> term1/1
  gnd1/1 -> out1/1
  gnd2/1 -> out2/1
  gnd/1 -> out/1

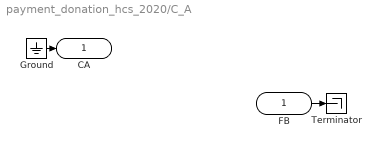
== system payment_donation_hcs_2020/C_A ==
  FB : Inport
      mask Display:
      | plot([0 60-10],[0 0]);
      | plot([0 0],[0 16]);
      | plot([0 60-10],[16 16]);
      | plot([60-10 60],[16 8]);
      | plot([60-10 60],[0 8]);
  Ground : Ground
  Terminator : Terminator
  CA : Outport
      mask Display:
      | plot([10 65],[0 0]);
      | plot([65-1 65-1],[0 16]);
      | plot([10 65],[16 16]);
      | plot([0 10],[8 16]);
      | plot([0 10],[8 0]);
  wires:
  Ground/1 -> CA/1
  FB/1 -> Terminator/1

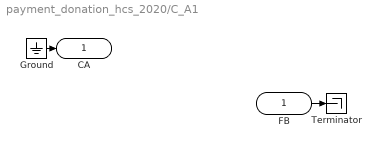
== system payment_donation_hcs_2020/C_A1 ==
  FB : Inport
      mask Display:
      | plot([0 60-10],[0 0]);
      | plot([0 0],[0 16]);
      | plot([0 60-10],[16 16]);
      | plot([60-10 60],[16 8]);
      | plot([60-10 60],[0 8]);
  Ground : Ground
  Terminator : Terminator
  CA : Outport
      mask Display:
      | plot([10 65],[0 0]);
      | plot([65-1 65-1],[0 16]);
      | plot([10 65],[16 16]);
      | plot([0 10],[8 16]);
      | plot([0 10],[8 0]);
  wires:
  FB/1 -> Terminator/1
  Ground/1 -> CA/1

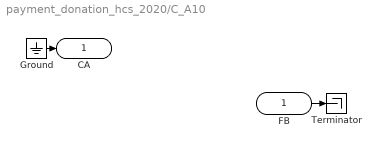
== system payment_donation_hcs_2020/C_A10 ==
  FB : Inport
      mask Display:
      | plot([0 60-10],[0 0]);
      | plot([0 0],[0 16]);
      | plot([0 60-10],[16 16]);
      | plot([60-10 60],[16 8]);
      | plot([60-10 60],[0 8]);
  Ground : Ground
  Terminator : Terminator
  CA : Outport
      mask Display:
      | plot([10 65],[0 0]);
      | plot([65-1 65-1],[0 16]);
      | plot([10 65],[16 16]);
      | plot([0 10],[8 16]);
      | plot([0 10],[8 0]);
  wires:
  Ground/1 -> CA/1
  FB/1 -> Terminator/1

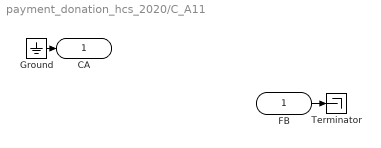
== system payment_donation_hcs_2020/C_A11 ==
  FB : Inport
      mask Display:
      | plot([0 60-10],[0 0]);
      | plot([0 0],[0 16]);
      | plot([0 60-10],[16 16]);
      | plot([60-10 60],[16 8]);
      | plot([60-10 60],[0 8]);
  Ground : Ground
  Terminator : Terminator
  CA : Outport
      mask Display:
      | plot([10 65],[0 0]);
      | plot([65-1 65-1],[0 16]);
      | plot([10 65],[16 16]);
      | plot([0 10],[8 16]);
      | plot([0 10],[8 0]);
  wires:
  Ground/1 -> CA/1
  FB/1 -> Terminator/1

== system payment_donation_hcs_2020/C_A2 ==
  FB : Inport
      mask Display:
      | plot([0 60-10],[0 0]);
      | plot([0 0],[0 16]);
      | plot([0 60-10],[16 16]);
      | plot([60-10 60],[16 8]);
      | plot([60-10 60],[0 8]);
  Ground : Ground
  Terminator : Terminator
  CA : Outport
      mask Display:
      | plot([10 65],[0 0]);
      | plot([65-1 65-1],[0 16]);
      | plot([10 65],[16 16]);
      | plot([0 10],[8 16]);
      | plot([0 10],[8 0]);
  wires:
  Ground/1 -> CA/1
  FB/1 -> Terminator/1

== system payment_donation_hcs_2020/C_A3 ==
  FB : Inport
      mask Display:
      | plot([0 60-10],[0 0]);
      | plot([0 0],[0 16]);
      | plot([0 60-10],[16 16]);
      | plot([60-10 60],[16 8]);
      | plot([60-10 60],[0 8]);
  Ground : Ground
  Terminator : Terminator
  CA : Outport
      mask Display:
      | plot([10 65],[0 0]);
      | plot([65-1 65-1],[0 16]);
      | plot([10 65],[16 16]);
      | plot([0 10],[8 16]);
      | plot([0 10],[8 0]);
  wires:
  Ground/1 -> CA/1
  FB/1 -> Terminator/1

== system payment_donation_hcs_2020/C_A4 ==
  FB : Inport
      mask Display:
      | plot([0 60-10],[0 0]);
      | plot([0 0],[0 16]);
      | plot([0 60-10],[16 16]);
      | plot([60-10 60],[16 8]);
      | plot([60-10 60],[0 8]);
  Ground : Ground
  Terminator : Terminator
  CA : Outport
      mask Display:
      | plot([10 65],[0 0]);
      | plot([65-1 65-1],[0 16]);
      | plot([10 65],[16 16]);
      | plot([0 10],[8 16]);
      | plot([0 10],[8 0]);
  wires:
  Ground/1 -> CA/1
  FB/1 -> Terminator/1

== system payment_donation_hcs_2020/C_A5 ==
  FB : Inport
      mask Display:
      | plot([0 60-10],[0 0]);
      | plot([0 0],[0 16]);
      | plot([0 60-10],[16 16]);
      | plot([60-10 60],[16 8]);
      | plot([60-10 60],[0 8]);
  Ground : Ground
  Terminator : Terminator
  CA : Outport
      mask Display:
      | plot([10 65],[0 0]);
      | plot([65-1 65-1],[0 16]);
      | plot([10 65],[16 16]);
      | plot([0 10],[8 16]);
      | plot([0 10],[8 0]);
  wires:
  FB/1 -> Terminator/1
  Ground/1 -> CA/1

== system payment_donation_hcs_2020/C_A6 ==
  FB : Inport
      mask Display:
      | plot([0 60-10],[0 0]);
      | plot([0 0],[0 16]);
      | plot([0 60-10],[16 16]);
      | plot([60-10 60],[16 8]);
      | plot([60-10 60],[0 8]);
  Ground : Ground
  Terminator : Terminator
  CA : Outport
      mask Display:
      | plot([10 65],[0 0]);
      | plot([65-1 65-1],[0 16]);
      | plot([10 65],[16 16]);
      | plot([0 10],[8 16]);
      | plot([0 10],[8 0]);
  wires:
  Ground/1 -> CA/1
  FB/1 -> Terminator/1

== system payment_donation_hcs_2020/C_A7 ==
  FB : Inport
      mask Display:
      | plot([0 60-10],[0 0]);
      | plot([0 0],[0 16]);
      | plot([0 60-10],[16 16]);
      | plot([60-10 60],[16 8]);
      | plot([60-10 60],[0 8]);
  Ground : Ground
  Terminator : Terminator
  CA : Outport
      mask Display:
      | plot([10 65],[0 0]);
      | plot([65-1 65-1],[0 16]);
      | plot([10 65],[16 16]);
      | plot([0 10],[8 16]);
      | plot([0 10],[8 0]);
  wires:
  FB/1 -> Terminator/1
  Ground/1 -> CA/1

== system payment_donation_hcs_2020/C_A8 ==
  FB : Inport
      mask Display:
      | plot([0 60-10],[0 0]);
      | plot([0 0],[0 16]);
      | plot([0 60-10],[16 16]);
      | plot([60-10 60],[16 8]);
      | plot([60-10 60],[0 8]);
  Ground : Ground
  Terminator : Terminator
  CA : Outport
      mask Display:
      | plot([10 65],[0 0]);
      | plot([65-1 65-1],[0 16]);
      | plot([10 65],[16 16]);
      | plot([0 10],[8 16]);
      | plot([0 10],[8 0]);
  wires:
  FB/1 -> Terminator/1
  Ground/1 -> CA/1

== system payment_donation_hcs_2020/C_A9 ==
  FB : Inport
      mask Display:
      | plot([0 60-10],[0 0]);
      | plot([0 0],[0 16]);
      | plot([0 60-10],[16 16]);
      | plot([60-10 60],[16 8]);
      | plot([60-10 60],[0 8]);
  Ground : Ground
  Terminator : Terminator
  CA : Outport
      mask Display:
      | plot([10 65],[0 0]);
      | plot([65-1 65-1],[0 16]);
      | plot([10 65],[16 16]);
      | plot([0 10],[8 16]);
      | plot([0 10],[8 0]);
  wires:
  Ground/1 -> CA/1
  FB/1 -> Terminator/1

== system payment_donation_hcs_2020/ES ==
  inp : Inport
  term : Terminator
  wires:
  inp/1 -> term/1

== system payment_donation_hcs_2020/F_B ==
  FB : Inport
      mask Display:
      | plot([0 60-10],[0 0]);
      | plot([0 0],[0 16]);
      | plot([0 60-10],[16 16]);
      | plot([60-10 60],[16 8]);
      | plot([60-10 60],[0 8]);
  Ground : Ground
  Terminator : Terminator
  CA : Outport
      mask Display:
      | plot([10 65],[0 0]);
      | plot([65-1 65-1],[0 16]);
      | plot([10 65],[16 16]);
      | plot([0 10],[8 16]);
      | plot([0 10],[8 0]);
  wires:
  FB/1 -> Terminator/1
  Ground/1 -> CA/1

== system payment_donation_hcs_2020/F_B1 ==
  FB : Inport
      mask Display:
      | plot([0 60-10],[0 0]);
      | plot([0 0],[0 16]);
      | plot([0 60-10],[16 16]);
      | plot([60-10 60],[16 8]);
      | plot([60-10 60],[0 8]);
  Ground : Ground
  Terminator : Terminator
  CA : Outport
      mask Display:
      | plot([10 65],[0 0]);
      | plot([65-1 65-1],[0 16]);
      | plot([10 65],[16 16]);
      | plot([0 10],[8 16]);
      | plot([0 10],[8 0]);
  wires:
  Ground/1 -> CA/1
  FB/1 -> Terminator/1

== system payment_donation_hcs_2020/F_B10 ==
  FB : Inport
      mask Display:
      | plot([0 60-10],[0 0]);
      | plot([0 0],[0 16]);
      | plot([0 60-10],[16 16]);
      | plot([60-10 60],[16 8]);
      | plot([60-10 60],[0 8]);
  Ground : Ground
  Terminator : Terminator
  CA : Outport
      mask Display:
      | plot([10 65],[0 0]);
      | plot([65-1 65-1],[0 16]);
      | plot([10 65],[16 16]);
      | plot([0 10],[8 16]);
      | plot([0 10],[8 0]);
  wires:
  FB/1 -> Terminator/1
  Ground/1 -> CA/1

== system payment_donation_hcs_2020/F_B2 ==
  FB : Inport
      mask Display:
      | plot([0 60-10],[0 0]);
      | plot([0 0],[0 16]);
      | plot([0 60-10],[16 16]);
      | plot([60-10 60],[16 8]);
      | plot([60-10 60],[0 8]);
  Ground : Ground
  Terminator : Terminator
  CA : Outport
      mask Display:
      | plot([10 65],[0 0]);
      | plot([65-1 65-1],[0 16]);
      | plot([10 65],[16 16]);
      | plot([0 10],[8 16]);
      | plot([0 10],[8 0]);
  wires:
  Ground/1 -> CA/1
  FB/1 -> Terminator/1

== system payment_donation_hcs_2020/F_B3 ==
  FB : Inport
      mask Display:
      | plot([0 60-10],[0 0]);
      | plot([0 0],[0 16]);
      | plot([0 60-10],[16 16]);
      | plot([60-10 60],[16 8]);
      | plot([60-10 60],[0 8]);
  Ground : Ground
  Terminator : Terminator
  CA : Outport
      mask Display:
      | plot([10 65],[0 0]);
      | plot([65-1 65-1],[0 16]);
      | plot([10 65],[16 16]);
      | plot([0 10],[8 16]);
      | plot([0 10],[8 0]);
  wires:
  Ground/1 -> CA/1
  FB/1 -> Terminator/1

== system payment_donation_hcs_2020/F_B4 ==
  FB : Inport
      mask Display:
      | plot([0 60-10],[0 0]);
      | plot([0 0],[0 16]);
      | plot([0 60-10],[16 16]);
      | plot([60-10 60],[16 8]);
      | plot([60-10 60],[0 8]);
  Ground : Ground
  Terminator : Terminator
  CA : Outport
      mask Display:
      | plot([10 65],[0 0]);
      | plot([65-1 65-1],[0 16]);
      | plot([10 65],[16 16]);
      | plot([0 10],[8 16]);
      | plot([0 10],[8 0]);
  wires:
  FB/1 -> Terminator/1
  Ground/1 -> CA/1

== system payment_donation_hcs_2020/F_B5 ==
  FB : Inport
      mask Display:
      | plot([0 60-10],[0 0]);
      | plot([0 0],[0 16]);
      | plot([0 60-10],[16 16]);
      | plot([60-10 60],[16 8]);
      | plot([60-10 60],[0 8]);
  Ground : Ground
  Terminator : Terminator
  CA : Outport
      mask Display:
      | plot([10 65],[0 0]);
      | plot([65-1 65-1],[0 16]);
      | plot([10 65],[16 16]);
      | plot([0 10],[8 16]);
      | plot([0 10],[8 0]);
  wires:
  FB/1 -> Terminator/1
  Ground/1 -> CA/1

== system payment_donation_hcs_2020/F_B6 ==
  FB : Inport
      mask Display:
      | plot([0 60-10],[0 0]);
      | plot([0 0],[0 16]);
      | plot([0 60-10],[16 16]);
      | plot([60-10 60],[16 8]);
      | plot([60-10 60],[0 8]);
  Ground : Ground
  Terminator : Terminator
  CA : Outport
      mask Display:
      | plot([10 65],[0 0]);
      | plot([65-1 65-1],[0 16]);
      | plot([10 65],[16 16]);
      | plot([0 10],[8 16]);
      | plot([0 10],[8 0]);
  wires:
  Ground/1 -> CA/1
  FB/1 -> Terminator/1

== system payment_donation_hcs_2020/F_B7 ==
  FB : Inport
      mask Display:
      | plot([0 60-10],[0 0]);
      | plot([0 0],[0 16]);
      | plot([0 60-10],[16 16]);
      | plot([60-10 60],[16 8]);
      | plot([60-10 60],[0 8]);
  Ground : Ground
  Terminator : Terminator
  CA : Outport
      mask Display:
      | plot([10 65],[0 0]);
      | plot([65-1 65-1],[0 16]);
      | plot([10 65],[16 16]);
      | plot([0 10],[8 16]);
      | plot([0 10],[8 0]);
  wires:
  Ground/1 -> CA/1
  FB/1 -> Terminator/1

== system payment_donation_hcs_2020/F_B8 ==
  FB : Inport
      mask Display:
      | plot([0 60-10],[0 0]);
      | plot([0 0],[0 16]);
      | plot([0 60-10],[16 16]);
      | plot([60-10 60],[16 8]);
      | plot([60-10 60],[0 8]);
  Ground : Ground
  Terminator : Terminator
  CA : Outport
      mask Display:
      | plot([10 65],[0 0]);
      | plot([65-1 65-1],[0 16]);
      | plot([10 65],[16 16]);
      | plot([0 10],[8 16]);
      | plot([0 10],[8 0]);
  wires:
  FB/1 -> Terminator/1
  Ground/1 -> CA/1
